simulink library "utilities"  (R2025a)
settings: Solver=VariableStepAuto  StartTime=0.0  StopTime=10.0  RelTol=1e-3
values from neighbouring files (symbols this model uses):
  deltaAT = 37    [orbit_params.m]
  m = size(A, 2)    [wheel_analysis.m]
  omega_icrf2b_initial = [-0.3804;-0.2976;0.06] *0    [orbit_params.m]
  s = sign(h_bias)    [min_h.m]
  Ts = 0.1    [orbit_params.m]    (also in untitled2.m = 0.005)
undefined symbols (not defined in the file or in its folder): earth, gyro, IAU, Kalman, mag, mag_torque, moon, sigma_u, sigma_v, star, sun, wheel
libraries: simulink x17, aerolibutil x16, dspmathops x12, sharedutil x5, simulink_extras x5, matrix_library x4, $bdroot x4, dspstat3 x4, aerolibtransform2 x3
settings Model: Creator=OlguPilav  LastModifiedBy=OlguPilav

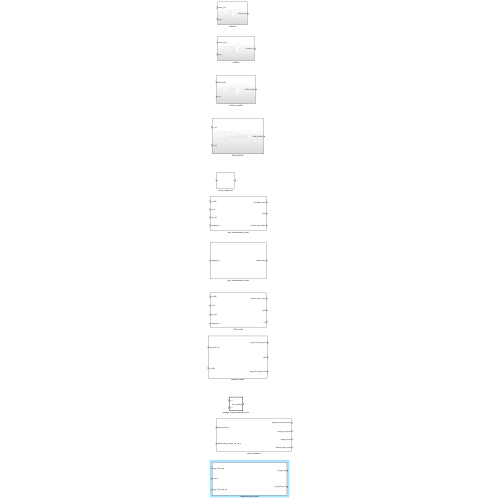
[thumbnail: Simulink's stored preview of the top-level diagram]
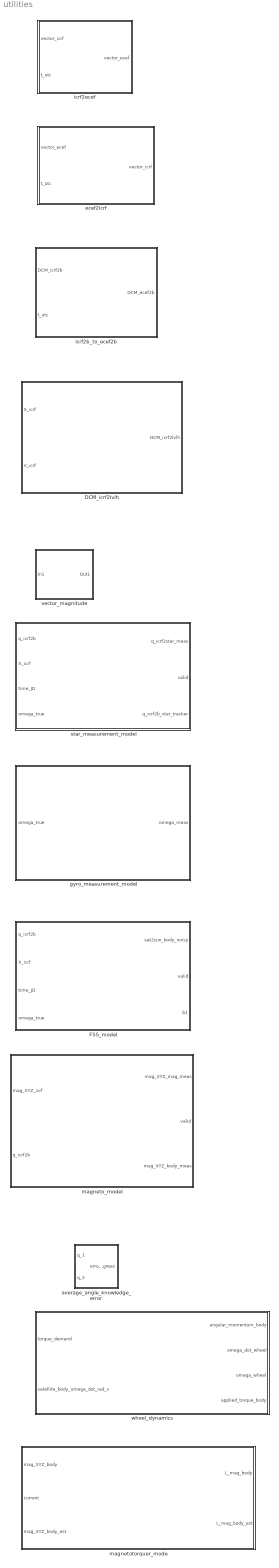
== system utilities ==
  DCM_icrf2lvlh : Subsystem
  FSS_model : Subsystem  mask{sun=sun}
  average_angle_knowledge_error : Subsystem  TreatAsAtomicUnit=on  SystemSampleTime=Kalman.Ts  mask{samples=10}
  ecef2icrf : Subsystem
  gyro_measurement_model : Subsystem  SystemSampleTime=Ts  mask{omega_initial=omega_icrf2b_initial, gyro=gyro}
  icrf2b_to_ecef2b : Subsystem
  icrf2ecef : Subsystem
  magneto_model : Subsystem  mask{mag=mag}
  magnetotorquer_mode : Subsystem  mask{Parameter1=mag_torque}
      mask prompts: Parameter1 "mag_torque"
      mask DialogControl mag_torque Prompt: mag_torque
  star_measurement_model : Subsystem  SystemSampleTime=Kalman.Ts  mask{star=star}
  vector_magnitude : Subsystem
  wheel_dynamics : Subsystem  mask{wheel=wheel, no=1}

== system utilities/DCM_icrf2lvlh ==
  X_icrf : Inport
  V_icrf : Inport  Port=2
  Cross Product : matrix_library/Cross Product
  Cross Product1 : matrix_library/Cross Product
  Gain : Gain  Gain=-1
  Matrix Concatenate : Concatenate  NumInputs=3  Mode=Multidimensional array
  Normalization : dspmathops/Normalization  NormType=2-norm  Bias=1e-10  NormOver=Each column  Dimension=1  roundingMode=Floor  overflowMode=off  accumDataTypeStr=Inherit: Same as product output  accumLastDataTypeStr=Inherit: Same as product output  outputDataTypeStr=Inherit: Same as product output  outputMin=[]  outputMax=[]  outputLastDataTypeStr=Inherit: Same as product output
  Normalization1 : dspmathops/Normalization  NormType=2-norm  Bias=1e-10  NormOver=Each column  Dimension=1  roundingMode=Floor  overflowMode=off  accumDataTypeStr=Inherit: Same as product output  accumLastDataTypeStr=Inherit: Same as product output  outputDataTypeStr=Inherit: Same as product output  outputMin=[]  outputMax=[]  outputLastDataTypeStr=Inherit: Same as product output
  Normalization2 : dspmathops/Normalization  NormType=2-norm  Bias=1e-10  NormOver=Each column  Dimension=1  roundingMode=Floor  overflowMode=off  accumDataTypeStr=Inherit: Same as product output  accumLastDataTypeStr=Inherit: Same as product output  outputDataTypeStr=Inherit: Same as product output  outputMin=[]  outputMax=[]  outputLastDataTypeStr=Inherit: Same as product output
  Transpose1 : Math  Operator=transpose
  Transpose2 : Math  Operator=transpose
  Transpose3 : Math  Operator=transpose
  DCM_icrf2lvlh : Outport
  wires:
  X_icrf/1 -> Normalization/1
  V_icrf/1 -> Normalization1/1
  Normalization/1 -> Cross Product/2, Gain/1
  Cross Product/1 -> Normalization2/1
  Transpose2/1 -> Matrix Concatenate/3
  Gain/1 -> Transpose2/1, Cross Product1/2  "z"
  Matrix Concatenate/1 -> DCM_icrf2lvlh/1
  Normalization2/1 -> Cross Product1/1, Transpose1/1
  Normalization1/1 -> Cross Product/1  "x"
  Transpose1/1 -> Matrix Concatenate/2
  Transpose3/1 -> Matrix Concatenate/1
  Cross Product1/1 -> Transpose3/1

== system utilities/FSS_model ==
  q_icrf2b : Inport
  X_icrf : Inport  Port=2  OutDataTypeStr=double  PortDimensions=3
  time_JD : Inport  Port=3  OutDataTypeStr=double  PortDimensions=1
  omega_true : Inport  Port=4  OutDataTypeStr=double  PortDimensions=3
  Equal : RelationalOperator  Operator=>  OutDataTypeStr=boolean  RndMeth=Simplest  InputSameDT=off
  NOT : Logic  Operator=NOT  IconShape=distinctive  AllPortsSameDT=off  OutDataTypeStr=boolean
  Subsystem : Subsystem  TreatAsAtomicUnit=on  SystemSampleTime=sun.Ts
  Unit Delay : UnitDelay  SampleTime=Kalman.Ts  HasFrameUpgradeWarning=on
  sat2sun_body_noisy : Outport
  valid : Outport  Port=2  OutDataTypeStr=boolean  SampleTime=[0.5,0]
  b1 : Outport  Port=3
  wires:
  Subsystem/3(tick) -> Equal/1, Unit Delay/1
  NOT/1 -> valid/1
  Subsystem/2(invalid) -> NOT/1  "invalid"
  time_JD/1 -> Subsystem/4(t_jd)  "t_utc"
  Unit Delay/1 -> Equal/2
  q_icrf2b/1 -> Subsystem/2(q_icrf2b)
  X_icrf/1 -> Subsystem/3(X_icrf)
  omega_true/1 -> Subsystem/1(omega_true)  "omega_icrf2b_b"
  Subsystem/1(sat2sun_body_noisy) -> sat2sun_body_noisy/1
  Subsystem/4(b1) -> b1/1

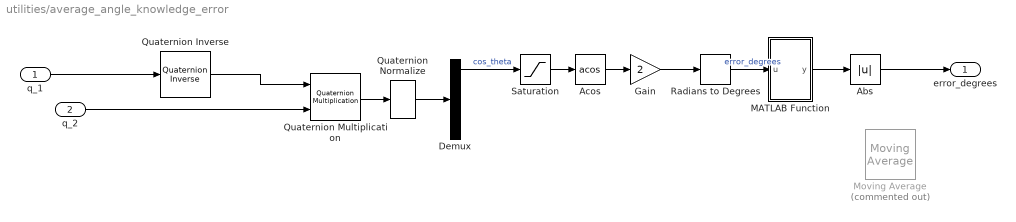
== system utilities/average_angle_knowledge_error ==
  q_1 : Inport
  q_2 : Inport  Port=2
  Abs : Abs  SaturateOnIntegerOverflow=off
  Acos : Trigonometry  Operator=acos
  Demux : Demux
  Gain : Gain  Gain=2
  MATLAB Function : MATLAB Function  TreatAsAtomicUnit=on
  Moving Average : dspstat3/Moving Average  Commented=on  Method=Sliding window  ForgettingFactorPort=off  SpecifyWindowLength=on  WindowLength=samples  OverlapLength=samples - 1  AllowArbitraryInputLength=off  ForgettingFactor=0.9  SimulateUsing=Interpreted execution
  Quaternion Inverse : aerolibutil/Quaternion Inverse
  Quaternion Multiplication : aerolibutil/Quaternion Multiplication
  Quaternion Normalize : sharedutil/Quaternion Normalize  aMode=aMode
  Radians to Degrees : simulink_extras/Transformations/Radians to Degrees
  Saturation : Saturate  UpperLimit=1  LowerLimit=-1
  error_degrees : Outport
  wires:
  q_1/1 -> Quaternion Inverse/1
  q_2/1 -> Quaternion Multiplication/2
  Quaternion Inverse/1 -> Quaternion Multiplication/1
  Quaternion Multiplication/1 -> Quaternion Normalize/1
  Demux/1 -> Saturation/1  "cos_theta"
  Radians to Degrees/1 -> MATLAB Function/1(u)  "error_degrees"
  Abs/1 -> error_degrees/1
  Quaternion Normalize/1 -> Demux/1
  Saturation/1 -> Acos/1
  Acos/1 -> Gain/1
  MATLAB Function/1(y) -> Abs/1
  Gain/1 -> Radians to Degrees/1

== system utilities/ecef2icrf ==
  vector_ecef : Inport
  t_utc : Inport  Port=2
  Clock : Clock  Commented=on
  Constant1 : Constant  Value=deltaAT
  Direction Cosine Matrix ECI to ECEF : aerolibtransform2/Direction Cosine Matrix ECI to ECEF  red=IAU-2000/2006  year=year  month=January  day=1  hour=hour  min=minute  sec=second  deltaT=None  errorflag=Error  extraparamflag=off
      settings: AttributesFormatString=%<red>
  Earth Orientation Parameters : EOParameters
  Matrix Multiply1 : Product  Multiplication=Matrix(*)
  Transpose : Math  Operator=transpose
  vector_icrf : Outport
  wires:
  t_utc/1 -> Earth Orientation Parameters/1
  Clock/1 -> ?
  Direction Cosine Matrix ECI to ECEF/1 -> Transpose/1
  Earth Orientation Parameters/2 -> ?
  Constant1/1 -> ?
  Earth Orientation Parameters/1 -> ?
  Earth Orientation Parameters/3 -> ?
  vector_ecef/1 -> Matrix Multiply1/2
  Matrix Multiply1/1 -> vector_icrf/1
  Transpose/1 -> Matrix Multiply1/1

== system utilities/gyro_measurement_model ==
  omega_true : Inport  PortDimensions=[3,1]
  Terminator : Terminator
  update_meas : Subsystem  TreatAsAtomicUnit=on  SystemSampleTime=gyro.Ts
  omega_meas : Outport
  wires:
  update_meas/1(omega_meas) -> omega_meas/1
  omega_true/1 -> update_meas/1(omega_true)
  update_meas/2(bias_true) -> Terminator/1

== system utilities/icrf2b_to_ecef2b ==
  DCM_icrf2b : Inport
  t_utc : Inport  Port=2
  Clock : Clock
  Constant1 : Constant  Value=deltaAT
  Direction Cosine Matrix ECI to ECEF : aerolibtransform2/Direction Cosine Matrix ECI to ECEF  red=IAU-2000/2006  year=year  month=January  day=1  hour=hour  min=minute  sec=second  deltaT=Sec  errorflag=Error  extraparamflag=on
      settings: AttributesFormatString=%<red>
  Earth Orientation Parameters : EOParameters
  Matrix Multiply1 : Product  Multiplication=Matrix(*)
  Transpose : Math  Operator=transpose
  DCM_ecef2b : Outport
  wires:
  t_utc/1 -> Earth Orientation Parameters/1
  Clock/1 -> Direction Cosine Matrix ECI to ECEF/5
  Direction Cosine Matrix ECI to ECEF/1 -> Transpose/1
  Earth Orientation Parameters/2 -> Direction Cosine Matrix ECI to ECEF/3
  Constant1/1 -> Direction Cosine Matrix ECI to ECEF/2
  Earth Orientation Parameters/1 -> Direction Cosine Matrix ECI to ECEF/1
  Earth Orientation Parameters/3 -> Direction Cosine Matrix ECI to ECEF/4
  DCM_icrf2b/1 -> Matrix Multiply1/1
  Matrix Multiply1/1 -> DCM_ecef2b/1
  Transpose/1 -> Matrix Multiply1/2  "ecef2icrf"

== system utilities/icrf2ecef ==
  vector_icrf : Inport
  t_utc : Inport  Port=2
  Constant1 : Constant  Value=deltaAT
  Direction Cosine Matrix ECI to ECEF : aerolibtransform2/Direction Cosine Matrix ECI to ECEF  red=IAU-2000/2006  year=year  month=January  day=1  hour=hour  min=minute  sec=second  deltaT=None  errorflag=Error  extraparamflag=off
      settings: AttributesFormatString=%<red>
  Earth Orientation Parameters : EOParameters
  Matrix Multiply1 : Product  Multiplication=Matrix(*)
  vector_ecef : Outport
  wires:
  t_utc/1 -> Earth Orientation Parameters/1
  Direction Cosine Matrix ECI to ECEF/1 -> Matrix Multiply1/1
  Earth Orientation Parameters/2 -> ?
  Constant1/1 -> ?
  Earth Orientation Parameters/1 -> ?
  Earth Orientation Parameters/3 -> ?
  vector_icrf/1 -> Matrix Multiply1/2
  Matrix Multiply1/1 -> vector_ecef/1

== system utilities/magneto_model ==
  mag_XYZ_icrf : Inport
  q_icrf2b : Inport  Port=2
  Constant : Constant
  Constant6 : Constant  Value=mag.dcm_mag2b
  Equal : RelationalOperator  Operator=>  OutDataTypeStr=boolean  RndMeth=Simplest  InputSameDT=off
  Matrix Multiply4 : Product  Multiplication=Matrix(*)
  Subsystem : Subsystem  TreatAsAtomicUnit=on  SystemSampleTime=mag.Ts
  Unit Delay : UnitDelay  SampleTime=Kalman.Ts  HasFrameUpgradeWarning=on
  mag_XYZ_mag_meas : Outport
  valid : Outport  Port=2
  mag_XYZ_body_meas : Outport  Port=3
  wires:
  mag_XYZ_icrf/1 -> Subsystem/1(mag_XYZ_icrf)
  q_icrf2b/1 -> Subsystem/2(q_icrf2b)
  Equal/1 -> ?
  Unit Delay/1 -> Equal/2
  Subsystem/2(tick) -> Equal/1, Unit Delay/1
  Subsystem/1(mag_XYZ_mag_meas) -> Matrix Multiply4/2, mag_XYZ_mag_meas/1
  Constant6/1 -> Matrix Multiply4/1
  Matrix Multiply4/1 -> mag_XYZ_body_meas/1  "mag_XYZ_body"
  Constant/1 -> valid/1

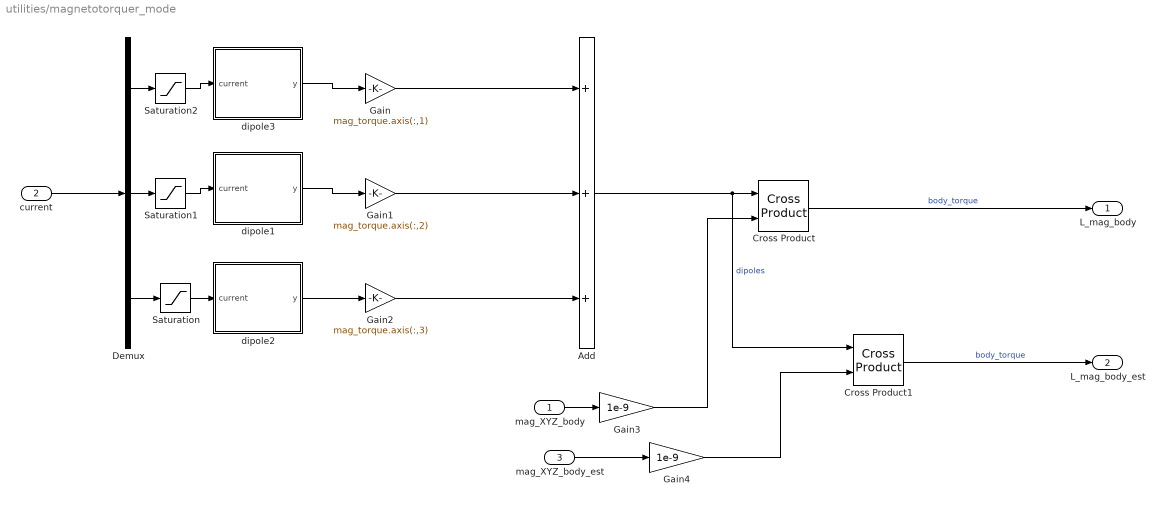
== system utilities/magnetotorquer_mode ==
  mag_XYZ_body : Inport
  current : Inport  Port=2
  mag_XYZ_body_est : Inport  Port=3
  Add : Sum  Inputs=+++
  Cross Product : matrix_library/Cross Product
  Cross Product1 : matrix_library/Cross Product
  Demux : Demux  Outputs=3
  Gain : Gain  Gain=mag_torque.axis(:,1)
  Gain1 : Gain  Gain=mag_torque.axis(:,2)
  Gain2 : Gain  Gain=mag_torque.axis(:,3)
  Gain3 : Gain  Gain=1e-9
  Gain4 : Gain  Gain=1e-9
  Saturation : Saturate  UpperLimit=mag_torque.I_max  LowerLimit=-mag_torque.I_max
  Saturation1 : Saturate  UpperLimit=mag_torque.I_max  LowerLimit=-mag_torque.I_max
  Saturation2 : Saturate  UpperLimit=mag_torque.I_max  LowerLimit=-mag_torque.I_max
  dipole1 : MATLAB Function  TreatAsAtomicUnit=on
  dipole2 : MATLAB Function  TreatAsAtomicUnit=on
  dipole3 : MATLAB Function  TreatAsAtomicUnit=on
  L_mag_body : Outport
  L_mag_body_est : Outport  Port=2
  wires:
  current/1 -> Demux/1
  Demux/1 -> Saturation2/1
  Demux/3 -> Saturation/1
  Demux/2 -> Saturation1/1
  dipole2/1(y) -> Gain2/1
  dipole1/1(y) -> Gain1/1
  dipole3/1(y) -> Gain/1
  Add/1 -> Cross Product1/1, Cross Product/1  "dipoles"
  mag_XYZ_body/1 -> Gain3/1
  Gain/1 -> Add/1
  Gain1/1 -> Add/2
  Gain2/1 -> Add/3
  Cross Product/1 -> L_mag_body/1  "body_torque"
  Gain3/1 -> Cross Product/2
  Saturation/1 -> dipole2/1(current)
  Saturation1/1 -> dipole1/1(current)
  Saturation2/1 -> dipole3/1(current)
  Cross Product1/1 -> L_mag_body_est/1  "body_torque"
  mag_XYZ_body_est/1 -> Gain4/1
  Gain4/1 -> Cross Product1/2

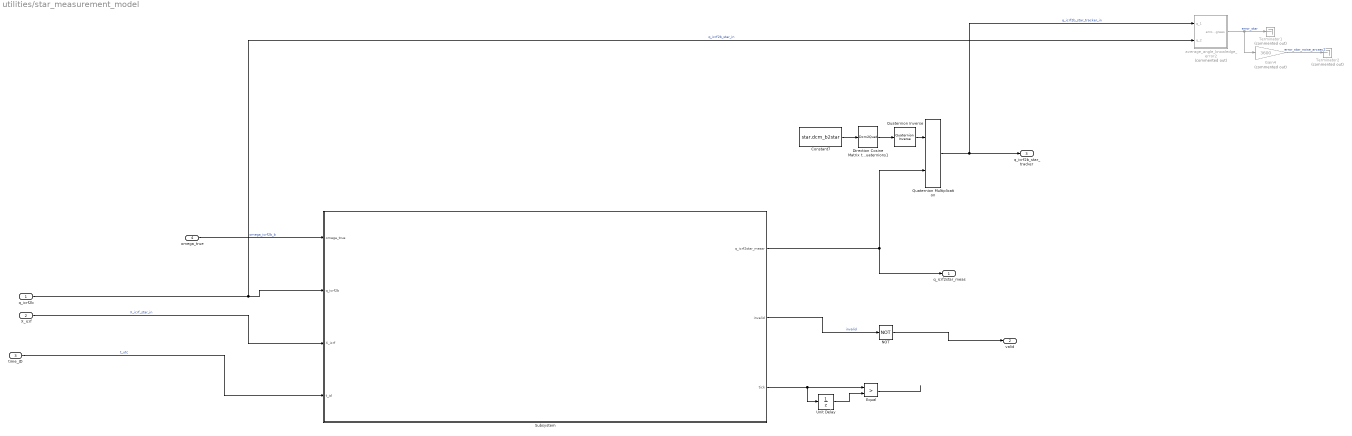
== system utilities/star_measurement_model ==
  q_icrf2b : Inport  OutDataTypeStr=double  PortDimensions=[4 1]
  X_icrf : Inport  Port=2  OutDataTypeStr=double  PortDimensions=3
  time_JD : Inport  Port=3  OutDataTypeStr=double  PortDimensions=1
  omega_true : Inport  Port=4  OutDataTypeStr=double  PortDimensions=3
  Constant7 : Constant  Value=star.dcm_b2star
  Direction Cosine Matrix to Quaternions1 : Dcm2Quat
  Equal : RelationalOperator  Operator=>  OutDataTypeStr=boolean  RndMeth=Simplest  InputSameDT=off
  Gain4 : Gain  Commented=on  Gain=3600
  NOT : Logic  Operator=NOT  IconShape=distinctive  AllPortsSameDT=off  OutDataTypeStr=boolean
  Quaternion Inverse : aerolibutil/Quaternion Inverse
  Quaternion Multiplication : aerolibutil/Quaternion Multiplication
  Subsystem : Subsystem  TreatAsAtomicUnit=on  SystemSampleTime=star.Ts
  Terminator1 : Terminator  Commented=on
  Terminator2 : Terminator  Commented=on
  Unit Delay : UnitDelay  SampleTime=Kalman.Ts  HasFrameUpgradeWarning=on
  average_angle_knowledge_error2 : Subsystem  Commented=on  AncestorBlock=utilities/star_measurement_model/Subsystem/average_angle_knowledge_error1  TreatAsAtomicUnit=on  SystemSampleTime=Kalman.Ts  mask{samples=2}
  q_icrf2star_meas : Outport  OutDataTypeStr=double  PortDimensions=4  SampleTime=[0.5,0]
  valid : Outport  Port=2  OutDataTypeStr=boolean  PortDimensions=1  SampleTime=[0.5,0]
  q_icrf2b_star_tracker : Outport  Port=3  OutDataTypeStr=double  PortDimensions=4  SampleTime=[0.5,0]
  wires:
  X_icrf/1 -> Subsystem/3(X_icrf)  "X_icrf_star_in"
  Quaternion Inverse/1 -> Quaternion Multiplication/1
  Subsystem/2(invalid) -> NOT/1  "invalid"
  Direction Cosine Matrix to Quaternions1/1 -> Quaternion Inverse/1
  q_icrf2b/1 -> average_angle_knowledge_error2/2(q_2), Subsystem/2(q_icrf2b)  "q_icrf2b_star_in"
  time_JD/1 -> Subsystem/4(t_jd)  "t_utc"
  Constant7/1 -> Direction Cosine Matrix to Quaternions1/1
  omega_true/1 -> Subsystem/1(omega_true)  "omega_icrf2b_b"
  Subsystem/1(q_icrf2star_measr) -> q_icrf2star_meas/1, Quaternion Multiplication/2
  Subsystem/3(tick) -> Unit Delay/1, Equal/1
  Unit Delay/1 -> Equal/2
  NOT/1 -> valid/1
  Equal/1 -> ?
  Gain4/1 -> Terminator2/1  "error_star_noise_arcsec2"
  Quaternion Multiplication/1 -> average_angle_knowledge_error2/1(q_1), q_icrf2b_star_tracker/1  "q_icrf2b_star_tracker_in"
  average_angle_knowledge_error2/1(error_degrees) -> Gain4/1, Terminator1/1  "error_star"

== system utilities/vector_magnitude ==
  In1 : Inport
  Dot Product2 : DotProduct  OutDataTypeStr=Inherit: Inherit via internal rule
  Sqrt2 : Sqrt
  Transpose3 : Math  Operator=transpose
  Out1 : Outport
  wires:
  Transpose3/1 -> Dot Product2/1
  Dot Product2/1 -> Sqrt2/1
  In1/1 -> Dot Product2/2, Transpose3/1
  Sqrt2/1 -> Out1/1

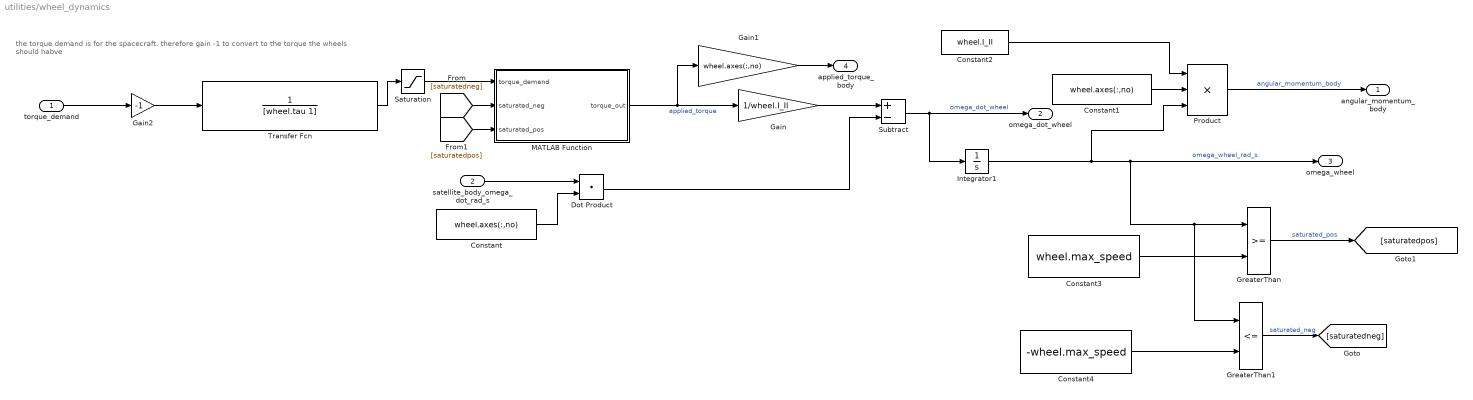
== system utilities/wheel_dynamics ==
  note: the torque demand is for the spacecraft. therefore gain -1 to convert to the torque the wheels should habve
  torque_demand : Inport
  satellite_body_omega_dot_rad_s : Inport  Port=2
  Constant : Constant  Value=wheel.axes(:,no)
  Constant1 : Constant  Value=wheel.axes(:,no)
  Constant2 : Constant  Value=wheel.I_II
  Constant3 : Constant  Value=wheel.max_speed
  Constant4 : Constant  Value=-wheel.max_speed
  Dot Product : DotProduct  OutDataTypeStr=Inherit: Inherit via internal rule
  Gain : Gain  Gain=1/wheel.I_II
  Gain1 : Gain  Gain=wheel.axes(:,no)
  Gain2 : Gain  Gain=-1
  GreaterThan : RelationalOperator  OutDataTypeStr=boolean  RndMeth=Simplest  InputSameDT=off
  GreaterThan1 : RelationalOperator  Operator=<=  OutDataTypeStr=boolean  RndMeth=Simplest  InputSameDT=off
  Integrator1 : Integrator  InitialCondition=wheel.omega_initial(no)
  MATLAB Function : MATLAB Function  TreatAsAtomicUnit=on
  Product : Product  Inputs=3
  Saturation : Saturate  UpperLimit=wheel.max_torque_Nm  LowerLimit=-wheel.max_torque_Nm
  Subtract : Sum  Inputs=+-
  Transfer Fcn : TransferFcn  Denominator=[wheel.tau 1]
  angular_momentum_body : Outport
  omega_dot_wheel : Outport  Port=2
  omega_wheel : Outport  Port=3
  applied_torque_body : Outport  Port=4
  wires:
  torque_demand/1 -> Gain2/1
  MATLAB Function/1(torque_out) -> Gain1/1, Gain/1  "applied_torque"
  satellite_body_omega_dot_rad_s/1 -> Dot Product/1
  Constant/1 -> Dot Product/2
  Gain/1 -> Subtract/1
  Dot Product/1 -> Subtract/2
  Subtract/1 -> Integrator1/1, omega_dot_wheel/1  "omega_dot_wheel"
  Product/1 -> angular_momentum_body/1  "angular_momentum_body"
  Gain1/1 -> applied_torque_body/1
  Constant1/1 -> Product/2
  Constant2/1 -> Product/1
  Transfer Fcn/1 -> Saturation/1
  Gain2/1 -> Transfer Fcn/1
  Constant3/1 -> GreaterThan/2
  Constant4/1 -> GreaterThan1/2
  Integrator1/1 -> Product/3, GreaterThan1/1, GreaterThan/1, omega_wheel/1  "omega_wheel_rad_s"
  Saturation/1 -> MATLAB Function/1(torque_demand)
  GreaterThan1/1 -> [saturatedneg]  "saturated_neg"
  [saturatedneg] -> MATLAB Function/2(saturated_neg)
  GreaterThan/1 -> [saturatedpos]  "saturated_pos"
  [saturatedpos] -> MATLAB Function/3(saturated_pos)

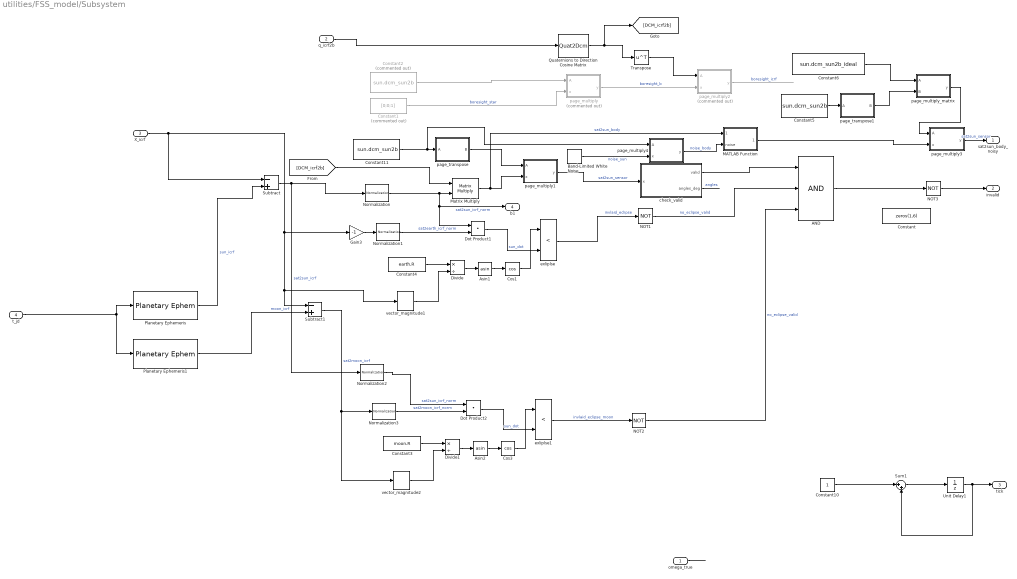
== system utilities/FSS_model/Subsystem ==
  omega_true : Inport
  q_icrf2b : Inport  Port=2
  X_icrf : Inport  Port=3
  t_jd : Inport  Port=4
  AND : Logic  Inputs=3  IconShape=distinctive  AllPortsSameDT=off  OutDataTypeStr=boolean
  Asin1 : Trigonometry  Operator=asin
  Asin2 : Trigonometry  Operator=asin
  Band-Limited White Noise : simulink/Sources/Band-Limited White Noise  Cov=sun.noise_unit * sun.sigma^2 * sun.Ts  Ts=sun.Ts  seed=sun.noise_seeds
  Constant : Constant  Value=zeros(1,6)
  Constant1 : Constant  Commented=on  Value=[0;0;1]
  Constant10 : Constant  OutDataTypeStr=uint64
  Constant11 : Constant  Value=sun.dcm_sun2b
  Constant2 : Constant  Commented=on  Value=sun.dcm_sun2b
  Constant3 : Constant  Value=moon.R
  Constant4 : Constant  Value=earth.R
  Constant5 : Constant  Value=sun.dcm_sun2b
  Constant6 : Constant  Value=sun.dcm_sun2b_ideal
  Cos1 : Trigonometry  Operator=cos
  Cos3 : Trigonometry  Operator=cos
  Divide : Product  Inputs=*/
  Divide1 : Product  Inputs=*/
  Dot Product1 : DotProduct  OutDataTypeStr=Inherit: Inherit via internal rule
  Dot Product2 : DotProduct  OutDataTypeStr=Inherit: Inherit via internal rule
  Gain3 : Gain  Gain=-1
  MATLAB Function : MATLAB Function  TreatAsAtomicUnit=on
  Matrix Multiply : Product  Multiplication=Matrix(*)
  NOT1 : Logic  Operator=NOT  IconShape=distinctive  AllPortsSameDT=off  OutDataTypeStr=boolean
  NOT2 : Logic  Operator=NOT  IconShape=distinctive  AllPortsSameDT=off  OutDataTypeStr=boolean
  NOT3 : Logic  Operator=NOT  IconShape=distinctive  AllPortsSameDT=off  OutDataTypeStr=boolean
  Normalization{,1..3} (4 alike) : dspmathops/Normalization  NormType=2-norm  Bias=1e-10  NormOver=Each column  Dimension=1  roundingMode=Floor  overflowMode=off  accumDataTypeStr=Inherit: Same as product output  accumLastDataTypeStr=Inherit: Same as product output  outputDataTypeStr=Inherit: Same as product output  outputMin=[]  outputMax=[]  outputLastDataTypeStr=Inherit: Same as product output
  Planetary Ephemeris : PlanetaryEphem  units=m,m/s  target=Sun  outputVelocity=off
  Planetary Ephemeris1 : PlanetaryEphem  units=m,m/s  outputVelocity=off
  Quaternions to Direction Cosine Matrix : Quat2Dcm
  Subtract : Sum  Inputs=-+
  Subtract1 : Sum  Inputs=-+
  Sum1 : Sum  Inputs=|++
  Transpose : Math  Operator=transpose
  Unit Delay1 : UnitDelay  InitialCondition=uint64(0)  SampleTime=-1  HasFrameUpgradeWarning=on
  check_valid : MATLAB Function  TreatAsAtomicUnit=on
  exliplse : RelationalOperator  Operator=<  OutDataTypeStr=boolean  RndMeth=Simplest  InputSameDT=off
  exliplse1 : RelationalOperator  Operator=<  OutDataTypeStr=boolean  RndMeth=Simplest  InputSameDT=off
  page_multiply : MATLAB Function  Commented=on  TreatAsAtomicUnit=on
  page_multiply1 : MATLAB Function  TreatAsAtomicUnit=on
  page_multiply2 : MATLAB Function  Commented=on  TreatAsAtomicUnit=on
  page_multiply3 : MATLAB Function  TreatAsAtomicUnit=on
  page_multiply4 : MATLAB Function  TreatAsAtomicUnit=on
  page_multiply_matrix : MATLAB Function  TreatAsAtomicUnit=on
  page_transpose : MATLAB Function  TreatAsAtomicUnit=on
  page_transpose1 : MATLAB Function  TreatAsAtomicUnit=on
  vector_magnitude1 : $bdroot/vector_magnitude
  vector_magnitude2 : $bdroot/vector_magnitude
  sat2sun_body_noisy : Outport
  invalid : Outport  Port=2
  tick : Outport  Port=3
  b1 : Outport  Port=4
  wires:
  Unit Delay1/1 -> tick/1, Sum1/2
  Sum1/1 -> Unit Delay1/1
  Constant10/1 -> Sum1/1
  Constant1/1 -> page_multiply/2(x)  "boresight_star"
  Planetary Ephemeris/1 -> Subtract/2  "sun_icrf"
  X_icrf/1 -> vector_magnitude1/1, Subtract1/1, Gain3/1, Subtract/1
  page_multiply2/1(y) -> ?  "boresight_icrf"
  Planetary Ephemeris1/1 -> Subtract1/2  "moon_icrf"
  Quaternions to Direction Cosine Matrix/1 -> [DCM_icrf2b], Transpose/1
  Normalization/1 -> b1/1, Dot Product1/1, Matrix Multiply/2  "sat2sun_icrf_norm"
  omega_true/1 -> ?
  Transpose/1 -> page_multiply2/1(A)
  q_icrf2b/1 -> Quaternions to Direction Cosine Matrix/1
  t_jd/1 -> Planetary Ephemeris/1, Planetary Ephemeris1/1
  page_multiply/1(y) -> page_multiply2/2(x)  "boresight_b"
  Constant2/1 -> page_multiply/1(A)
  Subtract1/1 -> vector_magnitude2/1, Normalization3/1  "sat2moon_icrf"
  [DCM_icrf2b] -> Matrix Multiply/1
  Matrix Multiply/1 -> MATLAB Function/1(sat2sun_body), page_multiply1/2(x)  "sat2sun_body"
  Constant11/1 -> page_multiply4/1(A), page_transpose/1(A)
  page_transpose/1(B) -> page_multiply1/1(A)
  page_multiply1/1(y) -> check_valid/1(x)  "sat2sun_sensor"
  check_valid/1(valid) -> AND/1
  check_valid/2(angles_deg) -> ?  "angles"
  Normalization1/1 -> Dot Product1/2  "sat2earth_icrf_norm"
  Gain3/1 -> Normalization1/1
  vector_magnitude1/1 -> Divide/2
  Divide/1 -> Asin1/1
  Constant4/1 -> Divide/1
  Dot Product1/1 -> exliplse/2  "sun_dot"
  exliplse/1 -> NOT1/1  "invlaid_eclipse"
  Asin1/1 -> Cos1/1
  Cos1/1 -> exliplse/1
  NOT1/1 -> AND/2  "no_eclipse_valid"
  AND/1 -> NOT3/1
  exliplse1/1 -> NOT2/1  "invlaid_eclipse_moon"
  Constant3/1 -> Divide1/1
  vector_magnitude2/1 -> Divide1/2
  Normalization3/1 -> Dot Product2/2  "sat2moon_icrf_norm"
  Subtract/1 -> Normalization2/1, Normalization/1  "sat2sun_icrf"
  Divide1/1 -> Asin2/1
  Cos3/1 -> exliplse1/1
  Dot Product2/1 -> exliplse1/2  "sun_dot"
  Asin2/1 -> Cos3/1
  Normalization2/1 -> Dot Product2/1  "sat2sun_icrf_norm"
  NOT2/1 -> AND/3  "no_eclipse_valid"
  Band-Limited White Noise/1 -> page_multiply4/2(x)  "noise_sun"
  MATLAB Function/1(noisy_meas) -> page_multiply3/2(x)
  NOT3/1 -> invalid/1
  Constant5/1 -> page_transpose1/1(A)
  page_transpose1/1(B) -> page_multiply_matrix/2(B)
  Constant6/1 -> page_multiply_matrix/1(A)
  page_multiply3/1(y) -> sat2sun_body_noisy/1  "sat2sun_sensor"
  page_multiply_matrix/1(y) -> page_multiply3/1(A)
  page_multiply4/1(y) -> MATLAB Function/2(noise)  "noise_body"

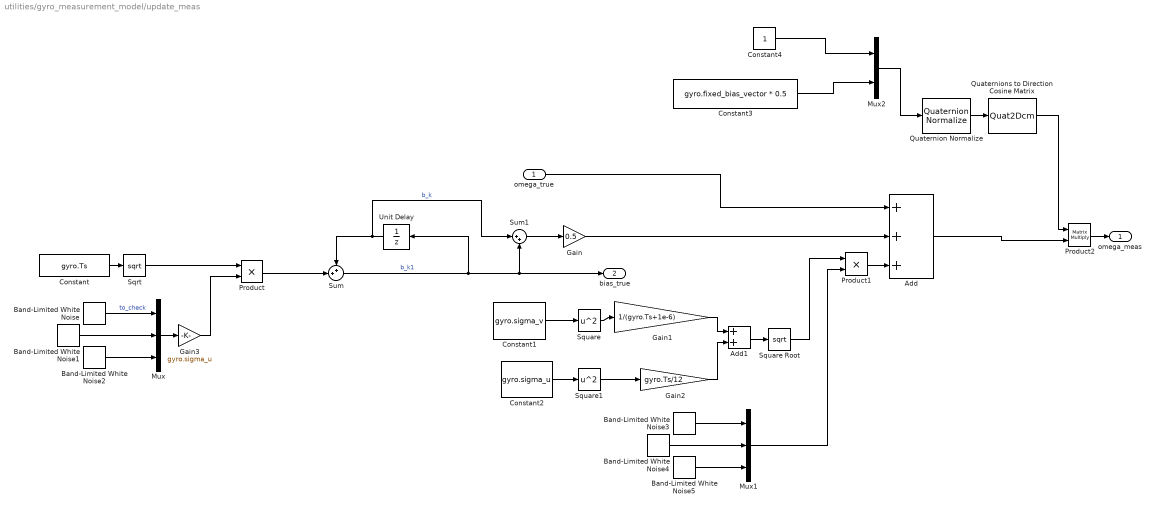
== system utilities/gyro_measurement_model/update_meas ==
  omega_true : Inport
  Add : Sum  Inputs=+++
  Add1 : Sum
  Band-Limited White Noise : simulink/Sources/Band-Limited White Noise  Cov=[gyro.Ts]  Ts=gyro.Ts  seed=[gyro.seed * 1]
  Band-Limited White Noise1 : simulink/Sources/Band-Limited White Noise  Cov=[gyro.Ts]  Ts=gyro.Ts  seed=gyro.seed * 2
  Band-Limited White Noise2 : simulink/Sources/Band-Limited White Noise  Cov=[gyro.Ts]  Ts=gyro.Ts  seed=gyro.seed * 3
  Band-Limited White Noise3 : simulink/Sources/Band-Limited White Noise  Cov=[gyro.Ts]  Ts=gyro.Ts  seed=gyro.seed * 4
  Band-Limited White Noise4 : simulink/Sources/Band-Limited White Noise  Cov=[gyro.Ts]  Ts=gyro.Ts  seed=gyro.seed * 5
  Band-Limited White Noise5 : simulink/Sources/Band-Limited White Noise  Cov=[gyro.Ts]  Ts=gyro.Ts  seed=gyro.seed * 6
  Constant : Constant  Value=gyro.Ts
  Constant1 : Constant  Value=gyro.sigma_v
  Constant2 : Constant  Value=gyro.sigma_u
  Constant3 : Constant  Value=gyro.fixed_bias_vector * 0.5
  Constant4 : Constant
  Gain : Gain  Gain=0.5
  Gain1 : Gain  Gain=1/(gyro.Ts+1e-6)
  Gain2 : Gain  Gain=gyro.Ts/12
  Gain3 : Gain  Gain=gyro.sigma_u
  Mux : Mux  Inputs=3
  Mux1 : Mux  Inputs=3
  Mux2 : Mux  Inputs=2
  Product : Product
  Product1 : Product
  Product2 : Product  Multiplication=Matrix(*)
  Quaternion Normalize : sharedutil/Quaternion Normalize  aMode=aMode
  Quaternions to Direction Cosine Matrix : Quat2Dcm
  Sqrt : Sqrt
  Square : Math  Operator=square
  Square Root : Sqrt
  Square1 : Math  Operator=square
  Sum : Sum  Inputs=++|
  Sum1 : Sum  Inputs=|++
  Unit Delay : UnitDelay  SampleTime=-1  HasFrameUpgradeWarning=on
  omega_meas : Outport
  bias_true : Outport  Port=2
  wires:
  Sum/1 -> Unit Delay/1, bias_true/1, Sum1/2  "b_k1"
  Unit Delay/1 -> Sum1/1, Sum/1  "b_k"
  Constant/1 -> Sqrt/1
  Band-Limited White Noise2/1 -> Mux/3
  Band-Limited White Noise1/1 -> Mux/2
  Band-Limited White Noise/1 -> Mux/1  "to_check"
  Product/1 -> Sum/2
  Sqrt/1 -> Product/1
  Mux/1 -> Gain3/1
  Sum1/1 -> Gain/1
  Add/1 -> Product2/2
  Gain/1 -> Add/2
  Band-Limited White Noise4/1 -> Mux1/2
  Mux1/1 -> Product1/2
  Band-Limited White Noise5/1 -> Mux1/3
  Band-Limited White Noise3/1 -> Mux1/1
  Product1/1 -> Add/3
  Constant1/1 -> Square/1
  Square/1 -> Gain1/1
  Constant2/1 -> Square1/1
  Square1/1 -> Gain2/1
  Gain1/1 -> Add1/1
  Gain2/1 -> Add1/2
  Add1/1 -> Square Root/1
  Square Root/1 -> Product1/1
  omega_true/1 -> Add/1
  Gain3/1 -> Product/2
  Constant3/1 -> Mux2/2
  Constant4/1 -> Mux2/1
  Mux2/1 -> Quaternion Normalize/1
  Quaternion Normalize/1 -> Quaternions to Direction Cosine Matrix/1
  Product2/1 -> omega_meas/1
  Quaternions to Direction Cosine Matrix/1 -> Product2/1

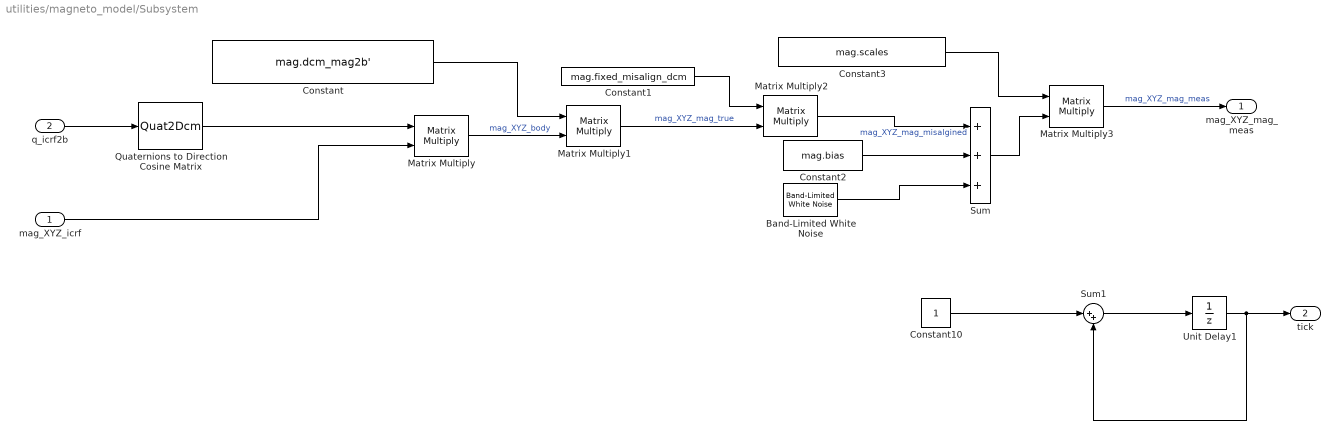
== system utilities/magneto_model/Subsystem ==
  mag_XYZ_icrf : Inport
  q_icrf2b : Inport  Port=2
  Band-Limited White Noise : simulink/Sources/Band-Limited White Noise  Cov=mag.co_var * mag.Ts  Ts=mag.Ts  seed=[mag.noise_seeds]
  Constant : Constant  Value=mag.dcm_mag2b'
  Constant1 : Constant  Value=mag.fixed_misalign_dcm
  Constant10 : Constant  OutDataTypeStr=uint64
  Constant2 : Constant  Value=mag.bias
  Constant3 : Constant  Value=mag.scales
  Matrix Multiply{,1..3} (4 alike) : Product  Multiplication=Matrix(*)
  Quaternions to Direction Cosine Matrix : Quat2Dcm
  Sum : Sum  Inputs=+++
  Sum1 : Sum  Inputs=|++
  Unit Delay1 : UnitDelay  InitialCondition=uint64(0)  SampleTime=-1  HasFrameUpgradeWarning=on
  mag_XYZ_mag_meas : Outport
  tick : Outport  Port=2
  wires:
  q_icrf2b/1 -> Quaternions to Direction Cosine Matrix/1
  Quaternions to Direction Cosine Matrix/1 -> Matrix Multiply/1
  mag_XYZ_icrf/1 -> Matrix Multiply/2
  Matrix Multiply/1 -> Matrix Multiply1/2  "mag_XYZ_body"
  Constant/1 -> Matrix Multiply1/1
  Matrix Multiply1/1 -> Matrix Multiply2/2  "mag_XYZ_mag_true"
  Constant1/1 -> Matrix Multiply2/1
  Matrix Multiply2/1 -> Sum/1  "mag_XYZ_mag_misalgined"
  Constant2/1 -> Sum/2
  Sum/1 -> Matrix Multiply3/2
  Constant3/1 -> Matrix Multiply3/1
  Matrix Multiply3/1 -> mag_XYZ_mag_meas/1  "mag_XYZ_mag_meas"
  Band-Limited White Noise/1 -> Sum/3
  Unit Delay1/1 -> tick/1, Sum1/2
  Constant10/1 -> Sum1/1
  Sum1/1 -> Unit Delay1/1

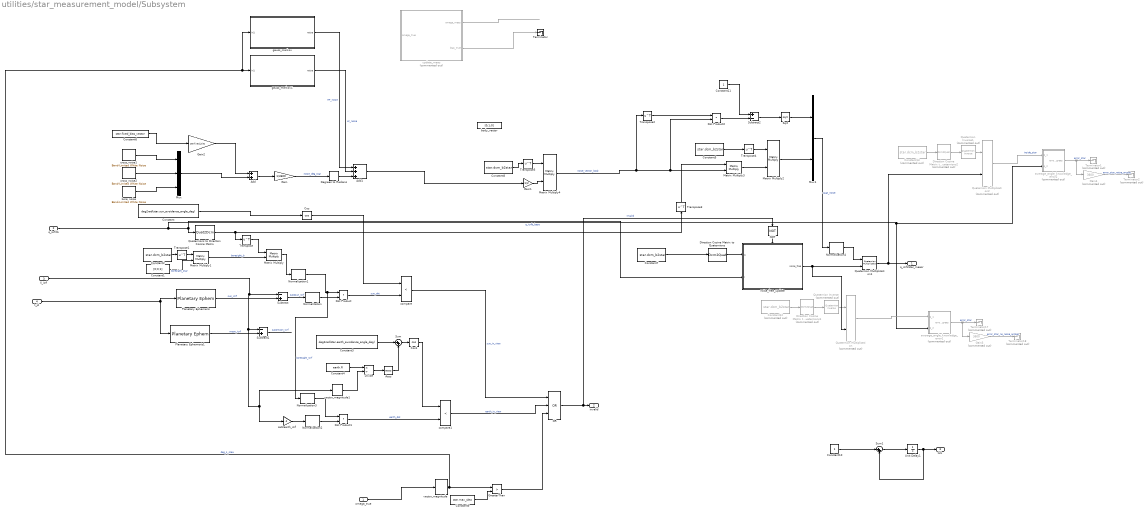
== system utilities/star_measurement_model/Subsystem ==
  omega_true : Inport
  q_icrf2b : Inport  Port=2
  X_icrf : Inport  Port=3
  t_jd : Inport  Port=4
  Acos : Trigonometry  Operator=acos
  Add : Sum
  Add1 : Sum  Inputs=+++
  Constant : Constant  Value=deg2rad(star.sun_avoidance_angle_deg)
  Constant1 : Constant  Value=[0;0;1]
  Constant10 : Constant  OutDataTypeStr=uint64
  Constant11 : Constant
  Constant12 : Constant  Commented=on  Value=star.dcm_b2star
  Constant13 : Constant  Commented=on  Value=star.dcm_b2star
  Constant{2,5,7..8} (4 alike) : Constant  Value=star.dcm_b2star
  Constant3 : Constant  Value=deg2rad(star.earth_avoidance_angle_deg)
  Constant4 : Constant  Value=earth.R
  Constant6 : Constant  Value=star.fixed_bias_vector
  Constant9 : Constant  Value=star.max_slew
  Cos : Trigonometry  Operator=cos
  Cos1 : Trigonometry  Operator=cos
  Degrees to Radians : simulink_extras/Transformations/Degrees to Radians
  Direction Cosine Matrix to Quaternions : Dcm2Quat
  Direction Cosine Matrix to Quaternions1 : Dcm2Quat  Commented=on
  Direction Cosine Matrix to Quaternions2 : Dcm2Quat  Commented=on
  Divide : Product  Inputs=*/
  Dot Product : DotProduct  OutDataTypeStr=Inherit: Inherit via internal rule
  Dot Product1 : DotProduct  OutDataTypeStr=Inherit: Inherit via internal rule
  Dot Product2 : DotProduct  OutDataTypeStr=Inherit: Inherit via internal rule
  Gain : Gain  Gain=1/3600
  Gain1 : Gain  Gain=1/2
  Gain2 : Gain  Gain=star.fixed_bias
  Gain3 : Gain  Commented=on  Gain=3600
  Gain4 : Gain  Commented=on  Gain=3600
  GreaterThan : RelationalOperator  Operator=>  OutDataTypeStr=boolean  RndMeth=Simplest  InputSameDT=off
  Matrix Multiply{,1..4} (5 alike) : Product  Multiplication=Matrix(*)
  Mux : Mux  Inputs=3
  Mux1 : Mux  Inputs=2
  NOT : Logic  Operator=NOT  IconShape=distinctive  AllPortsSameDT=off  OutDataTypeStr=boolean
  Normalization{,1..4} (5 alike) : dspmathops/Normalization  NormType=2-norm  Bias=1e-10  NormOver=Each column  Dimension=1  roundingMode=Floor  overflowMode=off  accumDataTypeStr=Inherit: Same as product output  accumLastDataTypeStr=Inherit: Same as product output  outputDataTypeStr=Inherit: Same as product output  outputMin=[]  outputMax=[]  outputLastDataTypeStr=Inherit: Same as product output
  OR : Logic  Operator=OR  Inputs=3  IconShape=distinctive  AllPortsSameDT=off  OutDataTypeStr=boolean
  Planetary Ephemeris : PlanetaryEphem  units=m,m/s  target=Sun  outputVelocity=off
  Planetary Ephemeris1 : PlanetaryEphem  units=m,m/s  outputVelocity=off
  Quaternion Inverse : aerolibutil/Quaternion Inverse  Commented=on
  Quaternion Inverse1 : aerolibutil/Quaternion Inverse  Commented=on
  Quaternion Multiplication : aerolibutil/Quaternion Multiplication  Commented=on
  Quaternion Multiplication1 : aerolibutil/Quaternion Multiplication
  Quaternion Multiplication2 : aerolibutil/Quaternion Multiplication  Commented=on
  Quaternions to Direction Cosine Matrix : Quat2Dcm
  Sqrt : Sqrt
  Subtract : Sum  Inputs=-+
  Subtract1 : Sum  Inputs=-+
  Subtract2 : Sum  Inputs=+-
  Sum : Sum  Inputs=|++
  Sum1 : Sum  Inputs=|++
  Terminator : Terminator
  Terminator{1..2,17..18} (4 alike) : Terminator  Commented=on
  Transpose{,1..5} (6 alike) : Math  Operator=transpose
  Unit Delay1 : UnitDelay  InitialCondition=uint64(0)  SampleTime=-1  HasFrameUpgradeWarning=on
  average_angle_knowledge_error1 : Subsystem  Commented=on  AncestorBlock=utilities/average_angle_knowledge_error  TreatAsAtomicUnit=on  SystemSampleTime=star.Ts  mask{samples=2}
  average_angle_knowledge_error2 : Subsystem  Commented=on  AncestorBlock=utilities/star_measurement_model/Subsystem/average_angle_knowledge_error1  TreatAsAtomicUnit=on  SystemSampleTime=star.Ts  mask{samples=2}
  body_vector : Constant  Value=[0;1;0]
  bore_noise : simulink/Sources/Band-Limited White Noise  Cov=[star.sigma_bore^2 * star.Ts]  Ts=star.Ts  seed=[star.seed * 3]
  compare : RelationalOperator  Operator=<  OutDataTypeStr=boolean  RndMeth=Simplest  InputSameDT=off
  compare1 : RelationalOperator  Operator=<  OutDataTypeStr=boolean  RndMeth=Simplest  InputSameDT=off
  cross_noise1 : simulink/Sources/Band-Limited White Noise  Cov=[star.sigma_cross^2 * star.Ts]  Ts=star.Ts  seed=[star.seed]
  cross_noise2 : simulink/Sources/Band-Limited White Noise  Cov=[star.sigma_cross^2 * star.Ts]  Ts=star.Ts  seed=[star.seed * 2]
  gauss_markov : Subsystem  mask{sigma=star.HF_sigma, def_tau=star.HF_def_tau}
  gauss_markov1 : Subsystem  AncestorBlock=utilities/star_measurement_model/Subsystem/gauss_markov  mask{sigma=star.LF_sigma, def_tau=star.LF_def_tau}
  noise_free_update : Subsystem
  sat2earth_icrf : Gain  Gain=-1
  update_meas : Subsystem  Commented=on  TreatAsAtomicUnit=on  SystemSampleTime=Ts
  vector_magnitude : $bdroot/vector_magnitude
  vector_magnitude1 : $bdroot/vector_magnitude
  q_icrf2star_measr : Outport
  invalid : Outport  Port=2
  tick : Outport  Port=3
  wires:
  Constant9/1 -> GreaterThan/2
  GreaterThan/1 -> OR/3
  NOT/1 -> noise_free_update/Enable
  Direction Cosine Matrix to Quaternions/1 -> noise_free_update/1(q)
  vector_magnitude/1 -> gauss_markov/1(In1), gauss_markov1/1(In1), GreaterThan/1  "deg_s_slew"
  Gain2/1 -> Add/1
  Constant6/1 -> Gain2/1
  Add/1 -> Gain/1
  Transpose5/1 -> Matrix Multiply4/1
  Constant8/1 -> Transpose5/1
  Matrix Multiply2/1 -> Mux1/2
  Transpose4/1 -> Matrix Multiply2/1
  Constant5/1 -> Transpose4/1
  Transpose3/1 -> Matrix Multiply3/1
  Matrix Multiply3/1 -> Matrix Multiply2/2
  Normalization4/1 -> Quaternion Multiplication1/1
  Matrix Multiply4/1 -> Dot Product2/2, Matrix Multiply3/2, Transpose2/1  "noise_vector_body"
  Subtract1/1 -> ?  "sat2moon_icrf"
  Gain/1 -> Degrees to Radians/1  "noise_deg_star"
  cross_noise1/1 -> Mux/1
  Dot Product1/1 -> compare1/2  "earth_dot"
  OR/1 -> invalid/1, NOT/1  "invalid"
  Normalization2/1 -> Dot Product1/2
  Normalization3/1 -> Dot Product1/1
  Transpose1/1 -> Matrix Multiply1/1
  Mux/1 -> Add/2
  Constant4/1 -> Divide/1
  Mux1/1 -> Normalization4/1  "quat_noise"
  Constant3/1 -> Sum/1
  Matrix Multiply1/1 -> Matrix Multiply/2  "boresight_b"
  vector_magnitude1/1 -> Divide/2
  Constant/1 -> Cos/1
  cross_noise2/1 -> Mux/2
  t_jd/1 -> Planetary Ephemeris1/1, Planetary Ephemeris/1
  Divide/1 -> Acos/1
  Constant7/1 -> Direction Cosine Matrix to Quaternions/1
  Matrix Multiply/1 -> Normalization1/1
  q_icrf2b/1 -> average_angle_knowledge_error2/2(q_2), average_angle_knowledge_error1/2(q_2), Quaternions to Direction Cosine Matrix/1, noise_free_update/2(r)  "q_icrfb_base"
  compare1/1 -> OR/2  "earth_in_view"
  Cos/1 -> compare/1
  compare/1 -> OR/1  "sun_in_view"
  Transpose/1 -> Matrix Multiply/1
  Subtract/1 -> Normalization/1  "sat2sun_icrf"
  Acos/1 -> Sum/2
  omega_true/1 -> vector_magnitude/1
  Normalization/1 -> Dot Product/2
  Cos1/1 -> compare1/1
  Quaternions to Direction Cosine Matrix/1 -> Transpose/1, Transpose3/1
  Constant2/1 -> Transpose1/1
  update_meas/2(bias_true) -> Terminator/1
  Planetary Ephemeris1/1 -> Subtract1/2  "moon_icrf"
  Normalization1/1 -> Dot Product/1, Normalization3/1  "boresight_icrf"
  update_meas/1(omega_meas) -> ?
  sat2earth_icrf/1 -> Normalization2/1
  Dot Product/1 -> compare/2  "sun_dot"
  Sqrt/1 -> Mux1/1
  X_icrf/1 -> Subtract/1, Subtract1/1, sat2earth_icrf/1, vector_magnitude1/1
  Sum/1 -> Cos1/1
  Planetary Ephemeris/1 -> Subtract/2  "sun_icrf"
  Constant1/1 -> Matrix Multiply1/2  "boresight_star"
  bore_noise/1 -> Mux/3
  Gain1/1 -> Matrix Multiply4/2
  Constant10/1 -> Sum1/1
  Sum1/1 -> Unit Delay1/1
  Unit Delay1/1 -> Sum1/2, tick/1
  Add1/1 -> Gain1/1
  Transpose2/1 -> Dot Product2/1
  Subtract2/1 -> Sqrt/1
  Dot Product2/1 -> Subtract2/2
  Constant11/1 -> Subtract2/1
  Quaternion Multiplication/1 -> average_angle_knowledge_error1/1(q_1)
  Gain3/1 -> Terminator18/1  "error_star_no_noise_arcsec"
  average_angle_knowledge_error1/1(error_degrees) -> Gain3/1, Terminator17/1  "error_star"
  Direction Cosine Matrix to Quaternions1/1 -> Quaternion Inverse/1
  Quaternion Inverse/1 -> Quaternion Multiplication/1
  Constant12/1 -> Direction Cosine Matrix to Quaternions1/1
  noise_free_update/1(noise_free) -> Quaternion Multiplication/2, Quaternion Multiplication1/2
  Quaternion Inverse1/1 -> Quaternion Multiplication2/1
  Quaternion Multiplication1/1 -> Quaternion Multiplication2/2, q_icrf2star_measr/1
  Direction Cosine Matrix to Quaternions2/1 -> Quaternion Inverse1/1
  Constant13/1 -> Direction Cosine Matrix to Quaternions2/1
  average_angle_knowledge_error2/1(error_degrees) -> Gain4/1, Terminator1/1  "error_star"
  Gain4/1 -> Terminator2/1  "error_star_noise_arcsec"
  Quaternion Multiplication2/1 -> average_angle_knowledge_error2/1(q_1)  "inside_star"
  gauss_markov/1(noise) -> Add1/1  "HF_noise"
  gauss_markov1/1(noise) -> Add1/2  "LF_noise"
  Degrees to Radians/1 -> Add1/3

== system utilities/star_measurement_model/average_angle_knowledge_error2 ==
  q_1 : Inport
  q_2 : Inport  Port=2
  Abs : Abs  SaturateOnIntegerOverflow=off
  Acos : Trigonometry  Operator=acos
  Demux : Demux
  MATLAB Function : MATLAB Function  TreatAsAtomicUnit=on
  Moving Average : dspstat3/Moving Average  Method=Sliding window  ForgettingFactorPort=off  SpecifyWindowLength=on  WindowLength=samples  OverlapLength=samples - 1  AllowArbitraryInputLength=off  ForgettingFactor=0.9  SimulateUsing=Interpreted execution
  Quaternion Inverse : aerolibutil/Quaternion Inverse
  Quaternion Multiplication : aerolibutil/Quaternion Multiplication
  Quaternion Normalize : sharedutil/Quaternion Normalize  aMode=aMode
  Radians to Degrees : simulink_extras/Transformations/Radians to Degrees
  Saturation : Saturate  UpperLimit=1  LowerLimit=-1
  error_degrees : Outport
  wires:
  q_1/1 -> Quaternion Inverse/1  "sd"
  q_2/1 -> Quaternion Multiplication/2  "sds"
  Quaternion Inverse/1 -> Quaternion Multiplication/1
  Quaternion Multiplication/1 -> Quaternion Normalize/1
  Demux/1 -> Saturation/1  "cos_theta"
  Radians to Degrees/1 -> MATLAB Function/1(u)  "error_degrees"
  Moving Average/1 -> error_degrees/1
  Abs/1 -> Moving Average/1
  Quaternion Normalize/1 -> Demux/1
  Saturation/1 -> Acos/1
  Acos/1 -> Radians to Degrees/1
  MATLAB Function/1(y) -> Abs/1

== system utilities/star_measurement_model/Subsystem/average_angle_knowledge_error1 ==
  q_1 : Inport
  q_2 : Inport  Port=2
  Abs : Abs  SaturateOnIntegerOverflow=off
  Acos : Trigonometry  Operator=acos
  Demux : Demux
  MATLAB Function : MATLAB Function  TreatAsAtomicUnit=on
  Moving Average : dspstat3/Moving Average  Method=Sliding window  ForgettingFactorPort=off  SpecifyWindowLength=on  WindowLength=samples  OverlapLength=samples - 1  AllowArbitraryInputLength=off  ForgettingFactor=0.9  SimulateUsing=Interpreted execution
  Quaternion Inverse : aerolibutil/Quaternion Inverse
  Quaternion Multiplication : aerolibutil/Quaternion Multiplication
  Quaternion Normalize : sharedutil/Quaternion Normalize  aMode=aMode
  Radians to Degrees : simulink_extras/Transformations/Radians to Degrees
  Saturation : Saturate  UpperLimit=1  LowerLimit=-1
  error_degrees : Outport
  wires:
  MATLAB Function/1(y) -> Abs/1
  Acos/1 -> Radians to Degrees/1
  Saturation/1 -> Acos/1
  Quaternion Normalize/1 -> Demux/1
  Abs/1 -> Moving Average/1
  Moving Average/1 -> error_degrees/1
  Radians to Degrees/1 -> MATLAB Function/1(u)  "error_degrees"
  Demux/1 -> Saturation/1  "cos_theta"
  Quaternion Multiplication/1 -> Quaternion Normalize/1
  Quaternion Inverse/1 -> Quaternion Multiplication/1
  q_2/1 -> Quaternion Multiplication/2
  q_1/1 -> Quaternion Inverse/1

== system utilities/star_measurement_model/Subsystem/average_angle_knowledge_error2 ==
  q_1 : Inport
  q_2 : Inport  Port=2
  Abs : Abs  SaturateOnIntegerOverflow=off
  Acos : Trigonometry  Operator=acos
  Demux : Demux
  MATLAB Function : MATLAB Function  TreatAsAtomicUnit=on
  Moving Average : dspstat3/Moving Average  Method=Sliding window  ForgettingFactorPort=off  SpecifyWindowLength=on  WindowLength=samples  OverlapLength=samples - 1  AllowArbitraryInputLength=off  ForgettingFactor=0.9  SimulateUsing=Interpreted execution
  Quaternion Inverse : aerolibutil/Quaternion Inverse
  Quaternion Multiplication : aerolibutil/Quaternion Multiplication
  Quaternion Normalize : sharedutil/Quaternion Normalize  aMode=aMode
  Radians to Degrees : simulink_extras/Transformations/Radians to Degrees
  Saturation : Saturate  UpperLimit=1  LowerLimit=-1
  error_degrees : Outport
  wires:
  q_1/1 -> Quaternion Inverse/1  "as"
  q_2/1 -> Quaternion Multiplication/2  "as"
  Quaternion Inverse/1 -> Quaternion Multiplication/1
  Quaternion Multiplication/1 -> Quaternion Normalize/1
  Demux/1 -> Saturation/1  "cos_theta"
  Radians to Degrees/1 -> MATLAB Function/1(u)  "error_degrees"
  Moving Average/1 -> error_degrees/1
  Abs/1 -> Moving Average/1
  Quaternion Normalize/1 -> Demux/1
  Saturation/1 -> Acos/1
  Acos/1 -> Radians to Degrees/1
  MATLAB Function/1(y) -> Abs/1

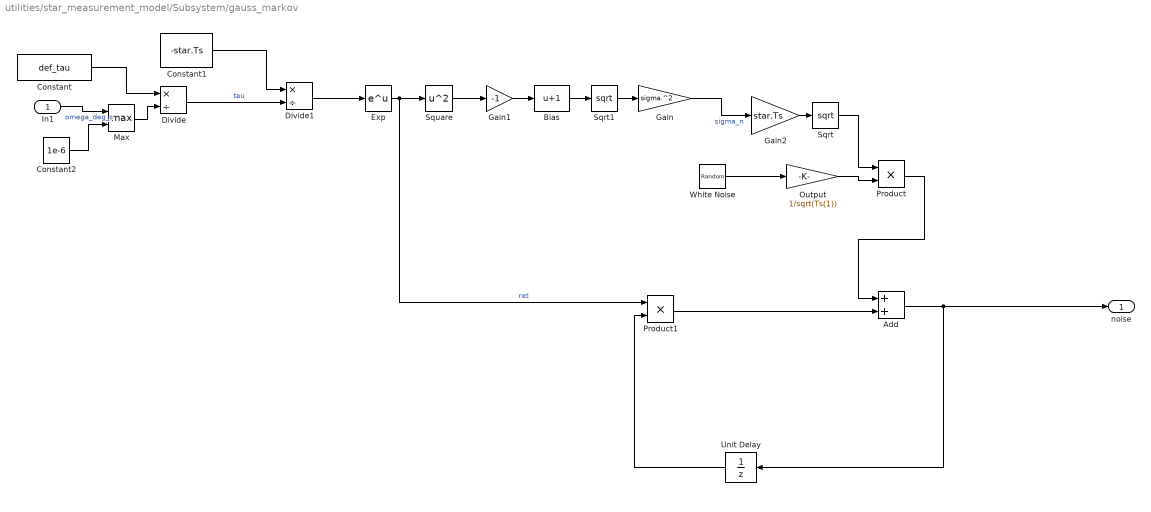
== system utilities/star_measurement_model/Subsystem/gauss_markov ==
  In1 : Inport
  Add : Sum
  Bias : Bias  Bias=1  SaturateOnIntegerOverflow=off
  Constant : Constant  Value=def_tau
  Constant1 : Constant  Value=-star.Ts
  Constant2 : Constant  Value=1e-6
  Divide : Product  Inputs=*/
  Divide1 : Product  Inputs=*/
  Exp : Math
  Gain : Gain  Gain=sigma.^2
  Gain1 : Gain  Gain=-1
  Gain2 : Gain  Gain=star.Ts
  Max : MinMax  Function=max  Inputs=2
  Output : Gain  Gain=1/sqrt(Ts(1))  SaturateOnIntegerOverflow=on  OutDataTypeStr=Inherit: Same as input  ParamDataTypeStr=Inherit: Same as input
  Product : Product
  Product1 : Product
  Sqrt : Sqrt
  Sqrt1 : Sqrt
  Square : Math  Operator=square
  Unit Delay : UnitDelay  SampleTime=-1  HasFrameUpgradeWarning=on
  White Noise : RandomNumber  DisableCoverage=on  Mean=[0,0,0]'  Variance=[1,1,1]'  Seed=[star.seed,star.seed+1,star.seed+2]  SampleTime=star.Ts
  noise : Outport
  wires:
  Add/1 -> Unit Delay/1, noise/1
  Product/1 -> Add/1
  Unit Delay/1 -> Product1/2
  Product1/1 -> Add/2
  White Noise/1 -> Output/1
  Output/1 -> Product/2
  Sqrt/1 -> Product/1
  In1/1 -> Max/1  "omega_deg_s"
  Gain2/1 -> Sqrt/1
  Constant/1 -> Divide/1
  Divide/1 -> Divide1/2  "tau"
  Constant1/1 -> Divide1/1
  Divide1/1 -> Exp/1
  Exp/1 -> Product1/1, Square/1  "ret"
  Square/1 -> Gain1/1
  Gain1/1 -> Bias/1
  Bias/1 -> Sqrt1/1
  Sqrt1/1 -> Gain/1
  Max/1 -> Divide/2
  Constant2/1 -> Max/2
  Gain/1 -> Gain2/1  "sigma_n"

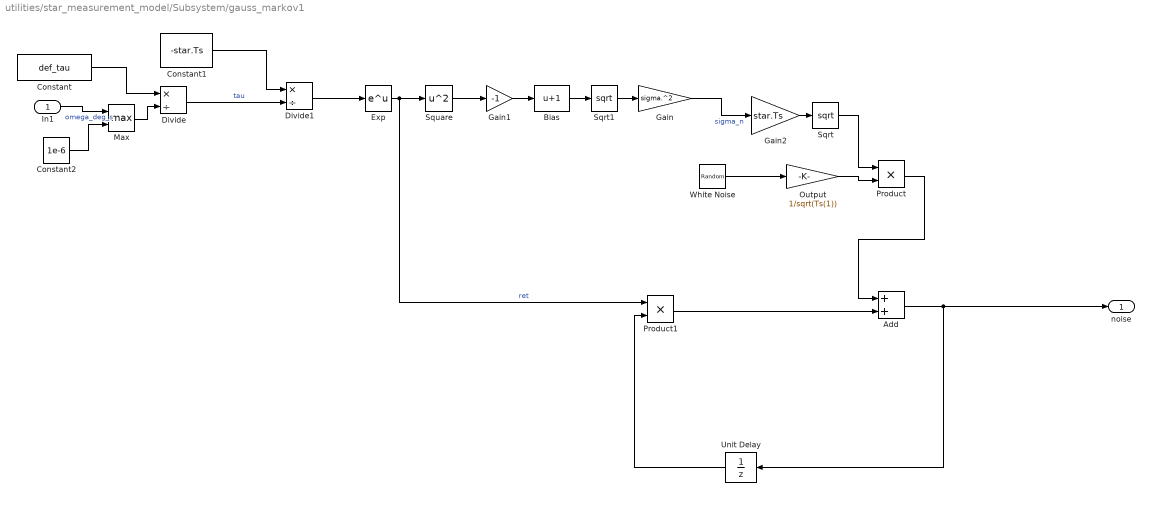
== system utilities/star_measurement_model/Subsystem/gauss_markov1 ==
  In1 : Inport
  Add : Sum
  Bias : Bias  Bias=1  SaturateOnIntegerOverflow=off
  Constant : Constant  Value=def_tau
  Constant1 : Constant  Value=-star.Ts
  Constant2 : Constant  Value=1e-6
  Divide : Product  Inputs=*/
  Divide1 : Product  Inputs=*/
  Exp : Math
  Gain : Gain  Gain=sigma.^2
  Gain1 : Gain  Gain=-1
  Gain2 : Gain  Gain=star.Ts
  Max : MinMax  Function=max  Inputs=2
  Output : Gain  Gain=1/sqrt(Ts(1))  SaturateOnIntegerOverflow=on  OutDataTypeStr=Inherit: Same as input  ParamDataTypeStr=Inherit: Same as input
  Product : Product
  Product1 : Product
  Sqrt : Sqrt
  Sqrt1 : Sqrt
  Square : Math  Operator=square
  Unit Delay : UnitDelay  SampleTime=-1  HasFrameUpgradeWarning=on
  White Noise : RandomNumber  DisableCoverage=on  Mean=[0,0,0]'  Variance=[1,1,1]'  Seed=[star.seed,star.seed+1,star.seed+2] *2  SampleTime=star.Ts
  noise : Outport
  wires:
  Gain/1 -> Gain2/1  "sigma_n"
  Constant2/1 -> Max/2
  Max/1 -> Divide/2
  Sqrt1/1 -> Gain/1
  Bias/1 -> Sqrt1/1
  Gain1/1 -> Bias/1
  Square/1 -> Gain1/1
  Exp/1 -> Square/1, Product1/1  "ret"
  Divide1/1 -> Exp/1
  Constant1/1 -> Divide1/1
  Divide/1 -> Divide1/2  "tau"
  Constant/1 -> Divide/1
  Gain2/1 -> Sqrt/1
  In1/1 -> Max/1  "omega_deg_s"
  Sqrt/1 -> Product/1
  Output/1 -> Product/2
  White Noise/1 -> Output/1
  Product1/1 -> Add/2
  Unit Delay/1 -> Product1/2
  Product/1 -> Add/1
  Add/1 -> noise/1, Unit Delay/1

== system utilities/star_measurement_model/Subsystem/noise_free_update ==
  q : Inport
  r : Inport  Port=2
  Enable : EnablePort
  Quaternion Multiplication : aerolibutil/Quaternion Multiplication
  noise_free : Outport
  wires:
  r/1 -> Quaternion Multiplication/2
  q/1 -> Quaternion Multiplication/1
  Quaternion Multiplication/1 -> noise_free/1  "noise_free"

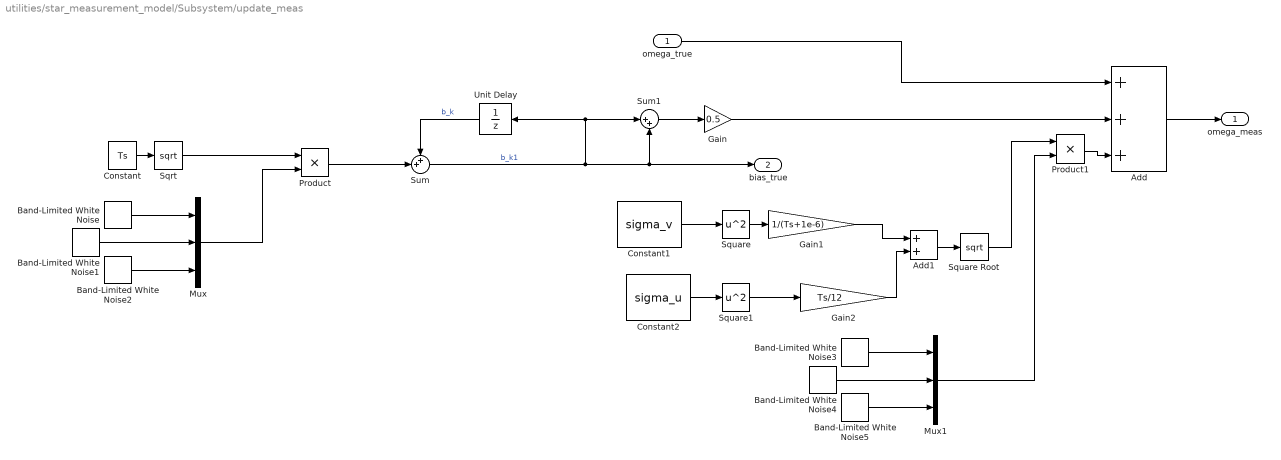
== system utilities/star_measurement_model/Subsystem/update_meas ==
  omega_true : Inport
  Add : Sum  Inputs=+++
  Add1 : Sum
  Band-Limited White Noise : simulink/Sources/Band-Limited White Noise  Cov=[Ts * sigma_u]  Ts=Ts  seed=[23341]
  Band-Limited White Noise1 : simulink/Sources/Band-Limited White Noise  Cov=[Ts * sigma_u]  Ts=Ts  seed=[2335341]
  Band-Limited White Noise2 : simulink/Sources/Band-Limited White Noise  Cov=[Ts * sigma_u]  Ts=Ts  seed=[231]
  Band-Limited White Noise3 : simulink/Sources/Band-Limited White Noise  Cov=[Ts * sigma_u]  Ts=Ts  seed=[23341]
  Band-Limited White Noise4 : simulink/Sources/Band-Limited White Noise  Cov=[Ts]  Ts=Ts  seed=[2335341]
  Band-Limited White Noise5 : simulink/Sources/Band-Limited White Noise  Cov=[Ts * sigma_u]  Ts=Ts  seed=[231]
  Constant : Constant  Value=Ts
  Constant1 : Constant  Value=sigma_v
  Constant2 : Constant  Value=sigma_u
  Gain : Gain  Gain=0.5
  Gain1 : Gain  Gain=1/(Ts+1e-6)
  Gain2 : Gain  Gain=Ts/12
  Mux : Mux  Inputs=3
  Mux1 : Mux  Inputs=3
  Product : Product
  Product1 : Product
  Sqrt : Sqrt
  Square : Math  Operator=square
  Square Root : Sqrt
  Square1 : Math  Operator=square
  Sum : Sum  Inputs=++|
  Sum1 : Sum  Inputs=|++
  Unit Delay : UnitDelay  SampleTime=-1  HasFrameUpgradeWarning=on
  omega_meas : Outport
  bias_true : Outport  Port=2
  wires:
  omega_true/1 -> Add/1
  Square Root/1 -> Product1/1
  Add1/1 -> Square Root/1
  Gain2/1 -> Add1/2
  Gain1/1 -> Add1/1
  Square1/1 -> Gain2/1
  Constant2/1 -> Square1/1
  Square/1 -> Gain1/1
  Constant1/1 -> Square/1
  Product1/1 -> Add/3
  Band-Limited White Noise3/1 -> Mux1/1
  Band-Limited White Noise5/1 -> Mux1/3
  Mux1/1 -> Product1/2
  Band-Limited White Noise4/1 -> Mux1/2
  Gain/1 -> Add/2
  Add/1 -> omega_meas/1
  Sum1/1 -> Gain/1
  Mux/1 -> Product/2
  Sqrt/1 -> Product/1
  Product/1 -> Sum/2
  Band-Limited White Noise/1 -> Mux/1
  Band-Limited White Noise1/1 -> Mux/2
  Band-Limited White Noise2/1 -> Mux/3
  Constant/1 -> Sqrt/1
  Unit Delay/1 -> Sum/1  "b_k"
  Sum/1 -> Sum1/2, bias_true/1, Unit Delay/1, Sum1/1  "b_k1"

== matlab function utilities/FSS_model/Subsystem/page_multiply2 ==
  data: A input; y output; x input
function y = f(A,x)
%#codegen
y = pagemtimes(A,x);

== matlab function utilities/star_measurement_model/Subsystem/average_angle_knowledge_error2/MATLAB Function ==
  data: u input; y output
function y = fcn(u)

if u < 0
    y = u + 180;
else
    y = u;
end

== matlab function utilities/FSS_model/Subsystem/page_multiply4 ==
  data: A input; y output; x input
function y = f(A,x)
%#codegen
y = pagemtimes(A,x);

== matlab function utilities/magnetotorquer_mode/dipole1 ==
  data: current input; y output; mag_torque parameter
function y = fcn(current, mag_torque)
y = (mag_torque.tanh_max * tanh(mag_torque.tanh_gain * current)) + mag_torque.residual;

== matlab function utilities/magnetotorquer_mode/dipole3 ==
  data: current input; y output; mag_torque parameter
function y = fcn(current, mag_torque)

y = (mag_torque.tanh_max * tanh(mag_torque.tanh_gain * current)) + mag_torque.residual;

== matlab function utilities/magnetotorquer_mode/dipole2 ==
  data: current input; y output; mag_torque parameter
function y = fcn(current, mag_torque)

y = (mag_torque.tanh_max * tanh(mag_torque.tanh_gain * current)) + mag_torque.residual;

== matlab function utilities/wheel_dynamics/MATLAB Function ==
  data: torque_demand input; torque_out output; saturated_neg input; saturated_pos input
function torque_out = fcn(torque_demand,saturated_neg,saturated_pos)

if saturated_pos
    torque_out = min(0,torque_demand);
elseif saturated_neg
    torque_out = max(0,torque_demand);
else
    torque_out = torque_demand;
end

== matlab function utilities/FSS_model/Subsystem/page_multiply ==
  data: A input; y output; x input
function y = f(A,x)
%#codegen
y = pagemtimes(A,x);

== matlab function utilities/FSS_model/Subsystem/check_valid ==
  data: valid output; angles_deg output; x input; sun parameter
function [valid,angles_deg] = f(x, sun)
angles_deg = zeros(2,1,length(x));
valid = boolean(zeros(1,6));

for k = 1:length(x)
    angles_deg(:,:,k) = [rad2deg(atan2(x(1,1,k),x(3,1,k)));rad2deg(atan2(x(2,1,k),x(3,1,k)))];
    valid(1,k) = ~(  abs(angles_deg(1,1,k)) > sun.FOV_half_angle_degrees || abs(angles_deg(2,1,k)) > sun.FOV_half_angle_degrees);

end

== matlab function utilities/FSS_model/Subsystem/page_multiply1 ==
  data: A input; y output; x input
function y = f(A,x)
%#codegen
y = pagemtimes(A,x);

== matlab function utilities/FSS_model/Subsystem/page_transpose ==
  data: A input; B output
function B = f(A)

B = pagetranspose(A);

== matlab function utilities/FSS_model/Subsystem/MATLAB Function ==
  data: sat2sun_body input; noisy_meas output; noise input
function noisy_meas = fcn(sat2sun_body,noise)

    matrix = repmat(sat2sun_body,[1,1,6]);
    noisy_meas = matrix + noise;
end

== matlab function utilities/average_angle_knowledge_error/MATLAB Function ==
  data: u input; y output
function y = fcn(u)

if u < 0
    y = u + 180;
else
    y = u;
end

if u > 180
    y = u - 360;
else
    y = u;
end

== matlab function utilities/FSS_model/Subsystem/page_multiply3 ==
  data: A input; y output; x input
function y = f(A,x)
%#codegen
y = pagemtimes(A,x);

== matlab function utilities/FSS_model/Subsystem/page_multiply_matrix ==
  data: A input; y output; B input
function y = f(A,B)
%#codegen
y = zeros(size(A));
for ii = 1:length(A)

    y(:,:,ii) = A(:,:,ii) * B(:,:,ii);
end

== matlab function utilities/FSS_model/Subsystem/page_transpose1 ==
  data: A input; B output
function B = f(A)

B = pagetranspose(A);

== matlab function utilities/star_measurement_model/Subsystem/average_angle_knowledge_error1/MATLAB Function ==
  data: u input; y output
function y = fcn(u)

if u < 0
    y = u + 180;
else
    y = u;
end

== matlab function utilities/star_measurement_model/average_angle_knowledge_error2/MATLAB Function ==
  data: u input; y output
function y = fcn(u)

if u < 0
    y = u + 180;
else
    y = u;
end
